simulink model "DIP_Model"  (R2021a)
settings: Solver=ode1  StartTime=0.0  StopTime=60  FixedStep=0.002  RelTol=1e-3  EnableMultiTasking=on
undefined symbols (not defined in the file): HIL, K, K_AMP, wcf_1, wcf_2, zetaf_1, zetaf_2
libraries: quarc_library x10, simulink_extras x7
settings Model: ExtModeTrigDuration=10000  Creator=Mechatronics  LastModifiedBy=User
settings SolverCC: AlgebraicLoopSolver=TrustRegion  PositivePriorityOrder=on
settings DataIOCC: ReturnWorkspaceOutputs=off
settings DebuggingCC: SFMachineParentedDataDiag=warning  ArithmeticOperatorsInVariantConditions=warning
settings SFSimCC: SimUseLocalCustomCode=off  CustomCodeUndefinedFunction=UseInterfaceOnly
settings RTWCC: Description=QUARC Win64 Target Using Toolchain  SystemTargetFile=quarc_win64.tlc  TemplateMakefile=quarc_default_tmf  RTWUseLocalCustomCode=off  Toolchain=QUARC win64 | nmake (64-bit Windows)  BuildConfiguration=Faster Runs
settings CodeAppCC: StateflowObjectComments=on
settings STFCustomTargetCC: TargetLangStandard=C99 (ISO)  ConcurrentExecutionCompliant=on  SystemTargetFile=quarc_win64.tlc
settings GRTTargetCC: ParMdlRefBuildCompliant=off  CompOptLevelCompliant=off  CombineOutputUpdateFcns=off  MatFileLogging=off  CPPClassGenCompliant=off  GRTInterface=on  ExtMode=on  ExtModeMexFile=quarc_comm
settings ConfigComp: CovMetricSettings=dswe

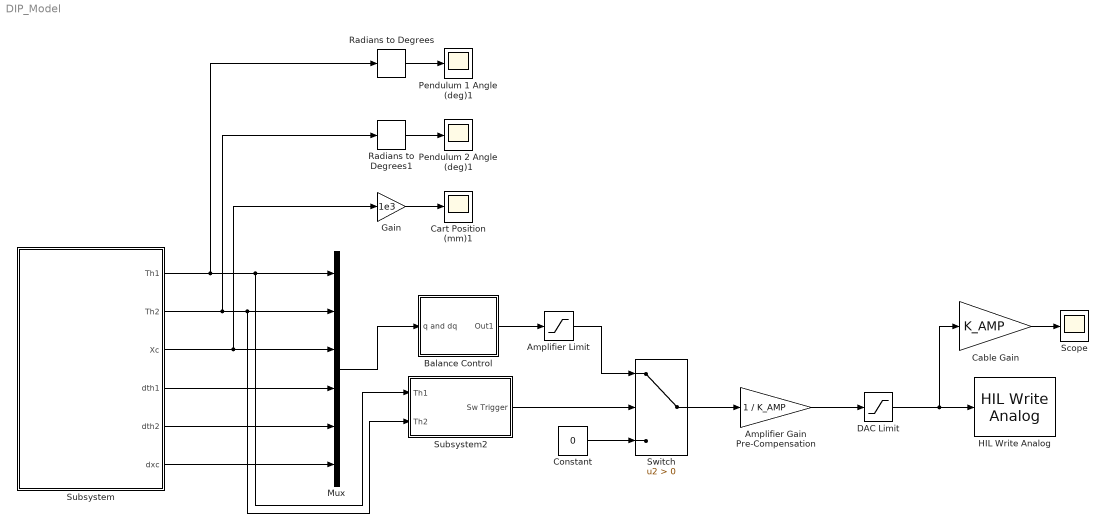
== system DIP_Model ==
  Amplifier Gain Pre-Compensation : Gain  Gain=1 / K_AMP  SaturateOnIntegerOverflow=on  OutDataTypeStr=Inherit: Same as input  ParamDataTypeStr=Inherit: Same as input
  Amplifier Limit : Saturate  UpperLimit=24  LowerLimit=-24
  Balance Control : Subsystem
  Cable Gain : Gain  Gain=K_AMP  SaturateOnIntegerOverflow=on  OutDataTypeStr=Inherit: Same as input  ParamDataTypeStr=Inherit: Same as input
  Cart Position (mm)1 : Scope
  Constant : Constant  Value=0
  DAC Limit : Saturate  UpperLimit=10  LowerLimit=-10
  Gain : Gain  Gain=1e3
  HIL Write Analog : quarc_library/Data Acquisition/Generic/Immediate I//O/HIL Write Analog  object_name=HIL-1  channels=0  sample_time=-1  active=off  vector_input=off
  Mux : Mux  Inputs=6
  Pendulum 1 Angle (deg)1 : Scope
  Pendulum 2 Angle (deg)1 : Scope
  Radians to Degrees : simulink_extras/Transformations/Radians to Degrees
  Radians to Degrees1 : simulink_extras/Transformations/Radians to Degrees
  Scope : Scope
  Subsystem : Subsystem
  Subsystem2 : Subsystem
  Switch : Switch  Criteria=u2 > Threshold
  wires:
  Subsystem/1(Th1) -> Radians to Degrees/1, Mux/1, Subsystem2/1(Th1)
  Subsystem/3(Xc) -> Gain/1, Mux/3
  Switch/1 -> Amplifier Gain Pre-Compensation/1
  Constant/1 -> Switch/3
  Cable Gain/1 -> Scope/1
  Subsystem/4(dth1) -> Mux/4
  Subsystem/2(Th2) -> Radians to Degrees1/1, Mux/2, Subsystem2/2(Th2)
  Subsystem/5(dth2) -> Mux/5
  Subsystem2/1(Sw Trigger) -> Switch/2
  Amplifier Limit/1 -> Switch/1
  Amplifier Gain Pre-Compensation/1 -> DAC Limit/1
  Balance Control/1(Out1) -> Amplifier Limit/1
  Gain/1 -> Cart Position (mm)1/1
  DAC Limit/1 -> Cable Gain/1, HIL Write Analog/1
  Subsystem/6(dxc) -> Mux/6
  Mux/1 -> Balance Control/1(q and dq)
  Radians to Degrees/1 -> Pendulum 1 Angle (deg)1/1
  Radians to Degrees1/1 -> Pendulum 2 Angle (deg)1/1

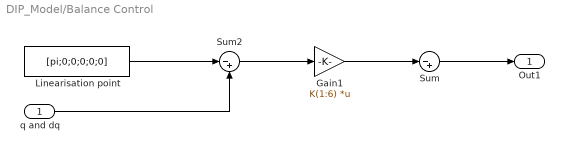
== system DIP_Model/Balance Control ==
  q and dq : Inport
  Gain1 : Gain  Gain=K(1:6)  Multiplication=Matrix(K*u)
  Linearisation point : Constant  Value=[pi;0;0;0;0;0]
  Sum : Sum  Inputs=|-+
  Sum2 : Sum  Inputs=|-+
  Out1 : Outport
  wires:
  Gain1/1 -> Sum/1
  Sum/1 -> Out1/1
  q and dq/1 -> Sum2/2
  Sum2/1 -> Gain1/1
  Linearisation point/1 -> Sum2/1

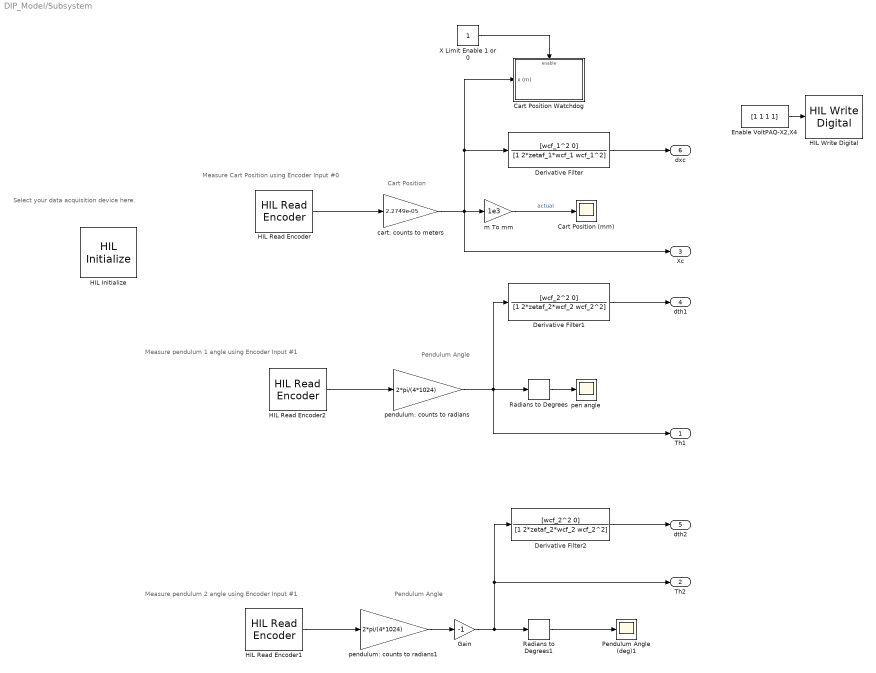
== system DIP_Model/Subsystem ==
  note: Measure Cart Position using Encoder Input #0
  note: Measure pendulum 1 angle using Encoder Input #1
  note: Pendulum Angle
  note: Cart Position
  note: Select your data acquisition device here.
  note: Pendulum Angle
  note: Measure pendulum 2 angle using Encoder Input #1
  Cart Position (mm) : Scope
  Cart Position Watchdog : Subsystem  TreatAsAtomicUnit=on
  Derivative Filter : TransferFcn  Numerator=[wcf_1^2 0]  Denominator=[1 2*zetaf_1*wcf_1 wcf_1^2]
  Derivative Filter1 : TransferFcn  Numerator=[wcf_2^2 0]  Denominator=[1 2*zetaf_2*wcf_2 wcf_2^2]
  Derivative Filter2 : TransferFcn  Numerator=[wcf_2^2 0]  Denominator=[1 2*zetaf_2*wcf_2 wcf_2^2]
  Enable VoltPAQ-X2,X4 : Constant  Value=[1 1 1 1]
  Gain : Gain  Gain=-1
  HIL Initialize : quarc_library/Data Acquisition/Generic/Configuration/HIL Initialize  object_name=HIL-1  board_type=q8_usb  board_number=0  board_options=update_rate=normal  exclusive=off  active=off  hardware_clocks=[0:2]  clock_modes=[]  initial_clock_frequencies=[]  set_clock_params_at_start=off  set_clock_params_at_switch_in=off  set_clock_frequencies_at_start=off  set_clock_frequencies_at_switch_in=off  analog_input_channels=[0:7]  analog_input_configurations=[]  analog_input_maximums=10  analog_input_minimums=-10  set_analog_input_params_at_start=on  set_analog_input_params_at_switch_in=off  analog_output_channels=[0:7]  analog_output_maximums=10  analog_output_minimums=-10  initial_analog_outputs=[0]  final_analog_outputs=[0]  watchdog_analog_outputs=0  set_analog_output_params_at_start=on  set_analog_output_params_at_switch_in=off  set_analog_outputs_at_start=on  set_analog_outputs_at_switch_in=off  set_analog_outputs_at_terminate=on  set_analog_outputs_at_switch_out=off  set_analog_outputs_on_watchdog=off  digital_input_channels=[]  digital_output_channels=[0:7]  digital_output_configuration=[]  initial_digital_outputs=[0]  final_digital_outputs=[0]  watchdog_digital_outputs=[0]  set_digital_output_params_at_start=off  set_digital_output_params_at_switch_in=off  set_digital_outputs_at_start=on  set_digital_outputs_at_switch_in=off  set_digital_outputs_at_terminate=on  set_digital_outputs_at_switch_out=off  set_digital_outputs_on_watchdog=off  encoder_channels=[0:7]  quadrature=[4]  encoder_filter_frequency=[]  initial_encoder_counts=[0]  set_encoder_params_at_start=on  set_encoder_params_at_switch_in=off  set_encoder_counts_at_start=on  set_encoder_counts_at_switch_in=off  pwm_channels=[0:7]  pwm_modes=0  pwm_frequency=99.532799999999995e6/4095  pwm_configuration=[0]  pwm_alignment=[0]  pwm_polarity=[1]  pwm_leading_deadband=[0]  pwm_trailing_deadband=[0]  initial_pwm_outputs=[0]  final_pwm_outputs=[0]  watchdog_pwm_outputs=[0]  set_pwm_params_at_start=on  set_pwm_params_at_switch_in=off  set_pwm_outputs_at_start=on  set_pwm_outputs_at_switch_in=off  set_pwm_outputs_at_terminate=on  set_pwm_outputs_at_switch_out=off  set_pwm_outputs_on_watchdog=off  other_output_channels=[]  initial_other_outputs=[]  final_other_outputs=[]  watchdog_other_outputs=[]  set_other_outputs_at_start=off  set_other_outputs_at_switch_in=off  set_other_outputs_at_terminate=off  set_other_outputs_at_switch_out=off  set_other_outputs_on_watchdog=off
  HIL Read Encoder : quarc_library/Data Acquisition/Generic/Immediate I//O/HIL Read Encoder  object_name=HIL-1  channels=[0]  sample_time=qc_get_step_size  active=on  vector_output=off  data_type_mode=Inherit via back propagation  data_type=double
  HIL Read Encoder1 : quarc_library/Data Acquisition/Generic/Immediate I//O/HIL Read Encoder  object_name=HIL-1  channels=[2]  sample_time=qc_get_step_size  active=on  vector_output=off  data_type_mode=Inherit via back propagation  data_type=double
  HIL Read Encoder2 : quarc_library/Data Acquisition/Generic/Immediate I//O/HIL Read Encoder  object_name=HIL-1  channels=[1]  sample_time=qc_get_step_size  active=on  vector_output=off  data_type_mode=Inherit via back propagation  data_type=double
  HIL Write Digital : quarc_library/Data Acquisition/Generic/Immediate I//O/HIL Write Digital  object_name=HIL-1  channels=[0:3]  sample_time=-1  active=off  vector_input=on
      settings: SourceProductName=QUARC Targets
  Pendulum Angle (deg)1 : Scope
  Radians to Degrees : simulink_extras/Transformations/Radians to Degrees
  Radians to Degrees1 : simulink_extras/Transformations/Radians to Degrees
  X Limit Enable 1 or 0 : Constant
  cart: counts to meters : Gain  Gain=2.2749e-05  SaturateOnIntegerOverflow=on  OutDataTypeStr=Inherit: Same as input  ParamDataTypeStr=Inherit: Same as input
  m To mm : Gain  Gain=1e3  SaturateOnIntegerOverflow=on  OutDataTypeStr=Inherit: Same as input  ParamDataTypeStr=Inherit: Same as input
  pen angle : Scope
  pendulum: counts to radians : Gain  Gain=2*pi/(4*1024)  SaturateOnIntegerOverflow=on  OutDataTypeStr=Inherit: Same as input  ParamDataTypeStr=Inherit: Same as input
  pendulum: counts to radians1 : Gain  Gain=2*pi/(4*1024)  SaturateOnIntegerOverflow=on  OutDataTypeStr=Inherit: Same as input  ParamDataTypeStr=Inherit: Same as input
  Th1 : Outport
  Th2 : Outport  Port=2
  Xc : Outport  Port=3
  dth1 : Outport  Port=4
  dth2 : Outport  Port=5
  dxc : Outport  Port=6
  wires:
  pendulum: counts to radians1/1 -> Gain/1
  pendulum: counts to radians/1 -> Radians to Degrees/1, Th1/1, Derivative Filter1/1
  m To mm/1 -> Cart Position (mm)/1  "actual"
  Radians to Degrees1/1 -> Pendulum Angle (deg)1/1
  HIL Read Encoder/1 -> cart: counts to meters/1
  Radians to Degrees/1 -> pen angle/1
  HIL Read Encoder2/1 -> pendulum: counts to radians/1
  HIL Read Encoder1/1 -> pendulum: counts to radians1/1
  Derivative Filter1/1 -> dth1/1
  Derivative Filter2/1 -> dth2/1
  Derivative Filter/1 -> dxc/1
  X Limit Enable 1 or 0/1 -> Cart Position Watchdog/Enable
  cart: counts to meters/1 -> Xc/1, Cart Position Watchdog/1(x (m)), Derivative Filter/1, m To mm/1
  Enable VoltPAQ-X2,X4/1 -> HIL Write Digital/1
  Gain/1 -> Radians to Degrees1/1, Th2/1, Derivative Filter2/1

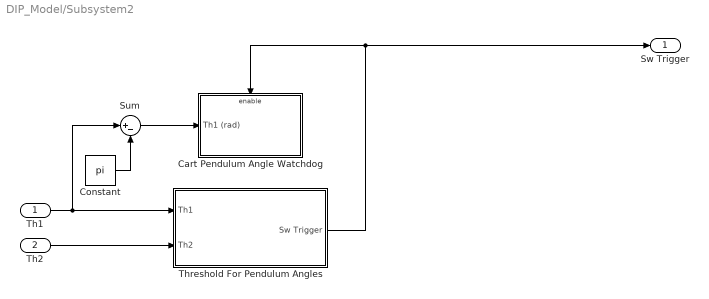
== system DIP_Model/Subsystem2 ==
  Th1 : Inport
  Th2 : Inport  Port=2
  Cart Pendulum Angle Watchdog : Subsystem  TreatAsAtomicUnit=on
  Constant : Constant  Value=pi
  Sum : Sum  Inputs=|+-
  Threshold For Pendulum Angles : Subsystem
  Sw Trigger : Outport
  wires:
  Th1/1 -> Sum/1, Threshold For Pendulum Angles/1(Th1)
  Threshold For Pendulum Angles/1(Sw Trigger) -> Sw Trigger/1, Cart Pendulum Angle Watchdog/Enable
  Th2/1 -> Threshold For Pendulum Angles/2(Th2)
  Sum/1 -> Cart Pendulum Angle Watchdog/1(Th1 (rad))
  Constant/1 -> Sum/2

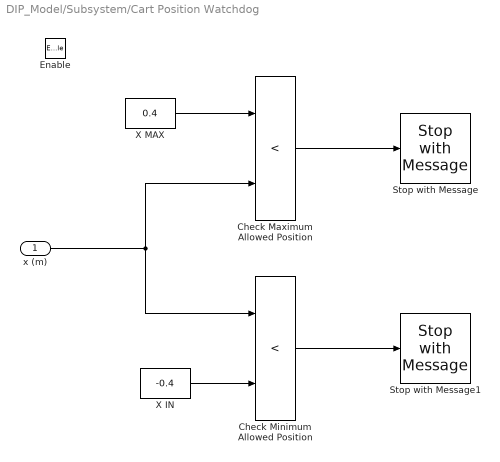
== system DIP_Model/Subsystem/Cart Position Watchdog ==
  x (m) : Inport
  Enable : EnablePort
  Check Maximum Allowed Position : RelationalOperator  Operator=<  RndMeth=Nearest  InputSameDT=on
  Check Minimum Allowed Position : RelationalOperator  Operator=<  RndMeth=Nearest  InputSameDT=on
  Stop with Message : quarc_library/Sinks/Error Handling/Stop with Message  message_type=Fixed error message  message_icon=Warning  message=Maximum Cart Limit Reached.
  Stop with Message1 : quarc_library/Sinks/Error Handling/Stop with Message  message_type=Fixed error message  message_icon=Warning  message=Minimum Cart Limit Reached.
  X IN : Constant  Value=-0.4
  X MAX : Constant  Value=0.4
  wires:
  X MAX/1 -> Check Maximum Allowed Position/1
  Check Minimum Allowed Position/1 -> Stop with Message1/1
  X IN/1 -> Check Minimum Allowed Position/2
  x (m)/1 -> Check Maximum Allowed Position/2, Check Minimum Allowed Position/1
  Check Maximum Allowed Position/1 -> Stop with Message/1

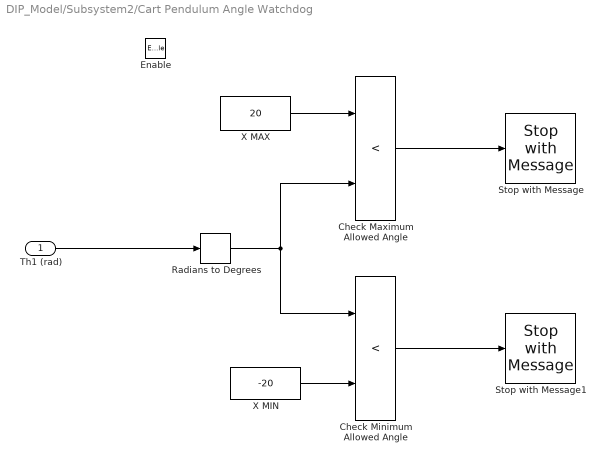
== system DIP_Model/Subsystem2/Cart Pendulum Angle Watchdog ==
  Th1 (rad) : Inport
  Enable : EnablePort
  Check Maximum Allowed Angle : RelationalOperator  Operator=<  RndMeth=Nearest  InputSameDT=on
  Check Minimum Allowed Angle : RelationalOperator  Operator=<  RndMeth=Nearest  InputSameDT=on
  Radians to Degrees : simulink_extras/Transformations/Radians to Degrees
  Stop with Message : quarc_library/Sinks/Error Handling/Stop with Message  message_type=Fixed error message  message_icon=Warning  message=Maximum Angle Reached for swing up.
  Stop with Message1 : quarc_library/Sinks/Error Handling/Stop with Message  message_type=Fixed error message  message_icon=Warning  message=Minimum Angle Reached for swing up.
  X MAX : Constant  Value=20
  X MIN : Constant  Value=-20
  wires:
  Radians to Degrees/1 -> Check Minimum Allowed Angle/1, Check Maximum Allowed Angle/2
  Check Maximum Allowed Angle/1 -> Stop with Message/1
  X MIN/1 -> Check Minimum Allowed Angle/2
  Check Minimum Allowed Angle/1 -> Stop with Message1/1
  X MAX/1 -> Check Maximum Allowed Angle/1
  Th1 (rad)/1 -> Radians to Degrees/1

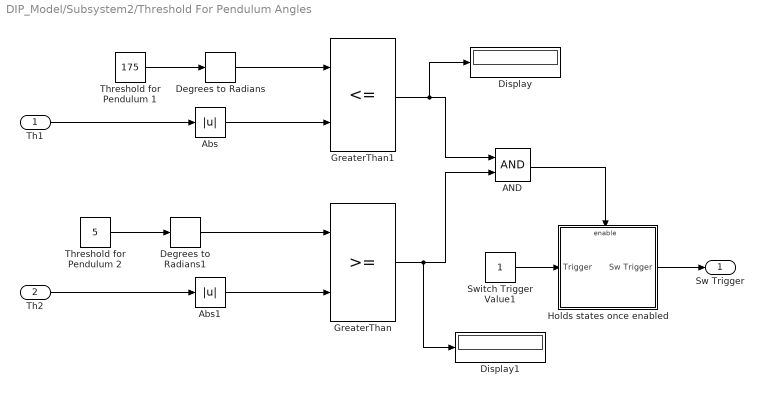
== system DIP_Model/Subsystem2/Threshold For Pendulum Angles ==
  Th1 : Inport
  Th2 : Inport  Port=2
  AND : Logic  AllPortsSameDT=off  OutDataTypeStr=boolean
  Abs : Abs
  Abs1 : Abs
  Degrees to Radians : simulink_extras/Transformations/Degrees to Radians
  Degrees to Radians1 : simulink_extras/Transformations/Degrees to Radians
  Display : Display
  Display1 : Display
  GreaterThan : RelationalOperator  OutDataTypeStr=boolean  RndMeth=Simplest
  GreaterThan1 : RelationalOperator  Operator=<=  OutDataTypeStr=boolean  RndMeth=Simplest
  Holds states once enabled : Subsystem  TreatAsAtomicUnit=on
  Switch Trigger Value1 : Constant
  Threshold for Pendulum 1 : Constant  Value=175
  Threshold for Pendulum 2 : Constant  Value=5
  Sw Trigger : Outport
  wires:
  Threshold for Pendulum 1/1 -> Degrees to Radians/1
  AND/1 -> Holds states once enabled/Enable
  GreaterThan1/1 -> Display/1, AND/1
  Threshold for Pendulum 2/1 -> Degrees to Radians1/1
  GreaterThan/1 -> Display1/1, AND/2
  Th1/1 -> Abs/1
  Th2/1 -> Abs1/1
  Holds states once enabled/1(Sw Trigger) -> Sw Trigger/1
  Abs1/1 -> GreaterThan/2
  Degrees to Radians1/1 -> GreaterThan/1
  Abs/1 -> GreaterThan1/2
  Degrees to Radians/1 -> GreaterThan1/1
  Switch Trigger Value1/1 -> Holds states once enabled/1(Trigger)

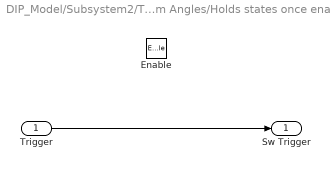
== system DIP_Model/Subsystem2/Threshold For Pendulum Angles/Holds states once enabled ==
  Trigger : Inport  OutDataTypeStr=double
  Enable : EnablePort
  Sw Trigger : Outport  OutDataTypeStr=double  InitialOutput=[0]
  wires:
  Trigger/1 -> Sw Trigger/1
